simulink model "Simu_LC_Case_II"  (R2018a)
settings: Solver=ode45  StartTime=0.0  StopTime=Map_Data.simu_time  RelTol=1e-3
values from neighbouring files (symbols this model uses):
  Map_Data = create_map(Global_Data)    [main.m]
undefined symbols (not defined in the file or in its folder): Auto
libraries: simulink x2, ModC_Planner x1, ModD_Controladores x1, ModG_Vehiculo x1
settings Model: Creator=Lisandro Cocca  LastModifiedBy=Lisandro Cocca

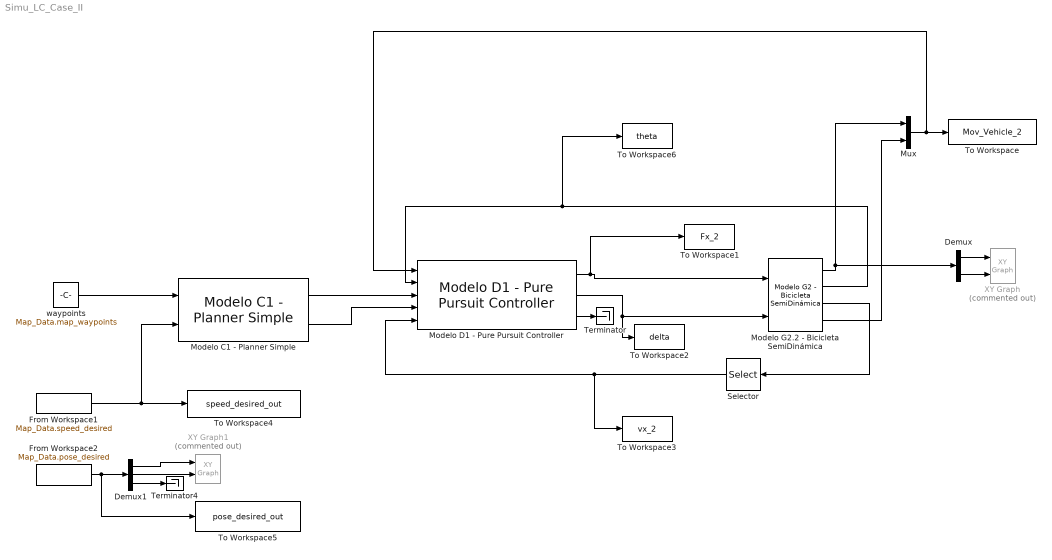
== system Simu_LC_Case_II ==
  Demux : Demux  Outputs=2
  Demux1 : Demux  Outputs=3
  From Workspace1 : FromWorkspace  VariableName=Map_Data.speed_desired  SampleTime=0  Interpolate=off  OutputAfterFinalValue=Setting to zero
  From Workspace2 : FromWorkspace  VariableName=Map_Data.pose_desired  SampleTime=0  Interpolate=off  OutputAfterFinalValue=Setting to zero
  Modelo C1 - Planner Simple : ModC_Planner/Modelo C1 - Planner Simple
      settings: SourceProductName=Proyecto_Final
  "Modelo D1 - Pure Pursuit Controller " : ModD_Controladores/Modelo D1 - Pure Pursuit Controller   kla=PP_Controller.kla  L=Auto.L  la_low=PP_Controller.la_low  psi_max=Auto.psi_max
      link override Memory1: InitialCondition=2200
      settings: SourceProductName=Proyecto_Final
  Modelo G2.2 - Bicicleta SemiDinámica : ModG_Vehiculo/Modelo G2 - Bicicleta SemiDinámica  L=Auto.L  m=Auto.m
      settings: SourceProductName=Proyecto_Final
  Mux : Mux  Inputs=2
  Selector : Selector  InputPortWidth=2  IndexOptions=Index vector (dialog)  Indices=[1]  OutputSizes=1
  Terminator : Terminator
  Terminator4 : Terminator
  To Workspace : ToWorkspace  VariableName=Mov_Vehicle_2  SampleTime=-1
  To Workspace1 : ToWorkspace  VariableName=Fx_2  SampleTime=-1
  To Workspace2 : ToWorkspace  VariableName=delta  SampleTime=-1
  To Workspace3 : ToWorkspace  VariableName=vx_2  SampleTime=-1
  To Workspace4 : ToWorkspace  VariableName=speed_desired_out  SampleTime=-1
  To Workspace5 : ToWorkspace  VariableName=pose_desired_out  SampleTime=-1
  To Workspace6 : ToWorkspace  VariableName=theta  SampleTime=-1
  XY Graph : simulink/Sinks/XY Graph  Commented=on  xmin=-20  xmax=20  ymin=-20  ymax=20  st=-1
  XY Graph1 : simulink/Sinks/XY Graph  Commented=on  xmin=-20  xmax=20  ymin=-20  ymax=20  st=-1
  "waypoints " : Constant  Value=Map_Data.map_waypoints  VectorParams1D=off
  wires:
  "Modelo D1 - Pure Pursuit Controller "/2 -> Modelo G2.2 - Bicicleta SemiDinámica/2, To Workspace2/1
  "Modelo D1 - Pure Pursuit Controller "/1 -> Modelo G2.2 - Bicicleta SemiDinámica/1, To Workspace1/1
  "waypoints "/1 -> Modelo C1 - Planner Simple/1
  From Workspace1/1 -> To Workspace4/1, Modelo C1 - Planner Simple/2
  Modelo C1 - Planner Simple/2 -> "Modelo D1 - Pure Pursuit Controller "/4
  Modelo C1 - Planner Simple/1 -> "Modelo D1 - Pure Pursuit Controller "/3
  From Workspace2/1 -> To Workspace5/1, Demux1/1
  Demux1/1 -> XY Graph1/1
  Demux1/2 -> XY Graph1/2
  Demux1/3 -> Terminator4/1
  Demux/1 -> XY Graph/1
  Demux/2 -> XY Graph/2
  Modelo G2.2 - Bicicleta SemiDinámica/1 -> Demux/1, Mux/1
  Mux/1 -> "Modelo D1 - Pure Pursuit Controller "/1, To Workspace/1
  Modelo G2.2 - Bicicleta SemiDinámica/2 -> To Workspace6/1, "Modelo D1 - Pure Pursuit Controller "/2
  Modelo G2.2 - Bicicleta SemiDinámica/4 -> Mux/2
  Modelo G2.2 - Bicicleta SemiDinámica/3 -> Selector/1
  Selector/1 -> To Workspace3/1, "Modelo D1 - Pure Pursuit Controller "/5
  "Modelo D1 - Pure Pursuit Controller "/3 -> Terminator/1
